simulink model "ValidateROM_PMSM"  (R2026a)
settings: Solver=FixedStepAuto  StartTime=0  StopTime=5000  FixedStep=0.5
PreLoadFcn:
  | % Load the Test data set for verification
  | load Data/pmsm_temperature_data_large.mat;
  | 
  | % Picking up a test profile for verification
  | TestSet = timetables{57};
  | 
  | % Seperate the predictors and the response
  | TestSet_Predict = TestSet(:,1:7);
  | TestSet_Response = TestSet(:,8:11);
  | 
  | % Clear the original data to avoid duplication
  | clear TestSet;
  | clear timetables;
  | 
  | % Load the trained LSTM and NSS Model
  | load Models/LSTMTrainingOutput.mat
  | load Models/NSSTrainingOutput.mat
  | 
  | % Extract the corresponding input normalizations
  | meanX_lstm = LSTMtrainingOutput.Normalization.Mu{1,1:7};
  | stdX_lstm = LSTMtrainingOutput.Normalization.Sigma{1,1:7};
  | 
  | meanX_nss = NSStrainingOutput.Normalization.Mu{1,1:7};
  | stdX_nss = NSStrainingOutput.Normalization.Sigma{1,1:7};
  | 
  | 
  | % Extract output normalization
  | meanY_lstm = LSTMtrainingOutput.Normalization.Mu{1,8:11};
  | stdY_lstm = LSTMtrainingOutput.Normalization.Sigma{1,8:11};
  | 
  | meanY_nss = NSStrainingOutput.Normalization.Mu{1,[8:11]};
  | stdY_nss = NSStrainingOutput.Normalization.Sigma{1,[8:11]};
  | 
  | %meanY_nss = NSStrainingOutput.Normalization.Mu{1,[8 11 14 17]};
  | %stdY_nss = NSStrainingOutput.Normalization.Sigma{1,[8 11 14 17]};
  | 
  | % [-1.4912 0 0 -1.0704 0 0 -1.2954 0 0 -1.3511 0 0]
model workspace (MAT data in the model file):
  time = -1
values from neighbouring files (symbols this model uses):
  NSStrainingOutput =     [NSSTrainingOutput.mat]
libraries: deeplib x1, slident x1
settings Model: Creator=skeshavm  LastModifiedBy=msatra
settings DataIOCC: SaveFormat=StructureWithTime
settings OptimizationCC: UseDivisionForNetSlopeComputation=on  GainParamInheritBuiltInType=on  UseFloatMulNetSlope=on  InlineInvariantSignals=on  StrengthReduction=on  PassReuseOutputArgsThreshold=0.0  InitFltsAndDblsToZero=on  EfficientFloat2IntCast=on  OptimizationPriority=Speed  MultiThreadedLoops=on  AutoScheduleForLoops=on  UseRestrictQualifier=on  DenormalBehavior=FlushToZero
settings DebuggingCC: InheritedTsInSrcMsg=none  MultiTaskCondExecSysMsg=none  MultiTaskRateTransMsg=warning
settings HardwareCC: TargetLongLongMode=on
settings SFSimCC: SimTargetLang=C++
settings RTWCC: Toolchain=Microsoft Visual C++ 2019 v16.0 | nmake (64-bit Windows)  BuildConfiguration=Faster Runs  TargetLang=C++  CheckMdlBeforeBuild=Warning  GPUErrorChecks=on  GPUComputeCapability=7.5
settings GRTTargetCC: TargetLangStandard=C++11 (ISO)  CodeInterfacePackaging=C++ class

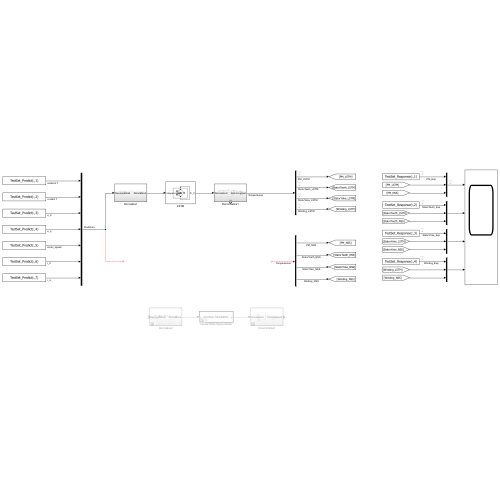
[thumbnail: Simulink's stored preview of the top-level diagram]
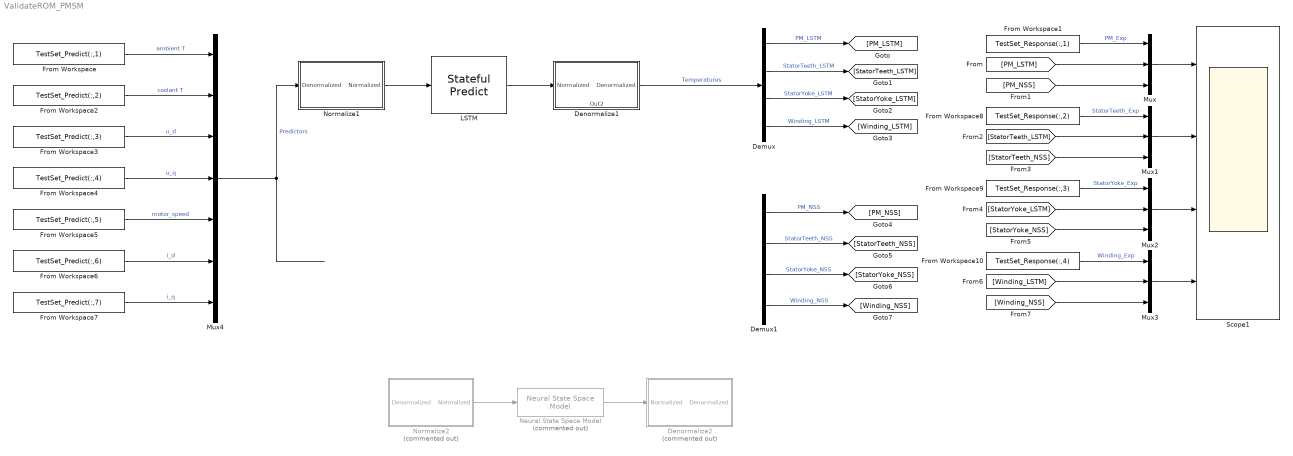
== system ValidateROM_PMSM ==
  Demux : Demux
  Demux1 : Demux
  Denormalize1 : Subsystem
      settings: PortSchema="{\"entries\":[{\"content\":{\"sides\":[{\"content\":{\"connectorIds\":[\"In1\"]},\"type\":\"ConnectorPlacement.EquallySpacedRectSide\",\"uuid\":\"378bcf4c-6683-4062-ab7f-3d581c01bba9\"},{\"content\":{\"connectorIds\":[\"Out1\"],\"side\":\"RIGHT\"},\"type\":\"ConnectorPlacement.EquallySpacedRectSide\",\"uuid\":\"d50369fd-00a0-4fa4-8ce4-c1bc44e9feeb\"},{\"content\":{\"side\":\"TOP\"},\"type\":\"ConnectorPlacement.EquallySpacedRectSide\",\"uuid\":\"bbe2daf0-7cf2-4950-af80-cb885b06a7dc\"},{\"content\":{\"connectorIds\":[\"Out2\"],\"side\":\"BOTTOM\"},\"type\":\"ConnectorPlacement.EquallySpacedRectSide\",\"uuid\":\"6647e6bb-1933-4f5d-ba46-5deef3c85e19\"}]},\"type\":\"ConnectorPlacement.EquallySpacedConnector\",\"uuid\":\"4ece9d1b-3b81-464e-b5f8-e83b248e3e90\"}],\"packageUris\":[\"http://schema.mathworks.com/mf0/Connector/R2020b\"],\"version\":\"1.0\"}"
  Denormalize2 : Subsystem  Commented=on
  From Workspace : FromWorkspace  VariableName=TestSet_Predict(:,1)
  From Workspace1 : FromWorkspace  VariableName=TestSet_Response(:,1)  SampleTime=5
  From Workspace10 : FromWorkspace  VariableName=TestSet_Response(:,4)  SampleTime=5
  From Workspace2 : FromWorkspace  VariableName=TestSet_Predict(:,2)
  From Workspace3 : FromWorkspace  VariableName=TestSet_Predict(:,3)
  From Workspace4 : FromWorkspace  VariableName=TestSet_Predict(:,4)
  From Workspace5 : FromWorkspace  VariableName=TestSet_Predict(:,5)
  From Workspace6 : FromWorkspace  VariableName=TestSet_Predict(:,6)
  From Workspace7 : FromWorkspace  VariableName=TestSet_Predict(:,7)
  From Workspace8 : FromWorkspace  VariableName=TestSet_Response(:,2)  SampleTime=5
  From Workspace9 : FromWorkspace  VariableName=TestSet_Response(:,3)  SampleTime=5
  LSTM : deeplib/Stateful Predict  Network=Network from MAT-file  NetworkFunction=untitled  NetworkFilePath=Models\LSTMTrainingNetwork.mat  SimulateUsing=Auto mode  InputDataFormats={ 'sequenceinput', 'CBT' }  SampleTime=0.5  ForceInterpretedSim=off  EnableDLNetwork=on  LastKnownNetworkFilePath=''  LastKnownNetworkTimeStamp=''
  Mux{,1..3} (4 alike) : Mux  Inputs=3
  Mux4 : Mux  Inputs=7
  Neural State Space Model : slident/Models/Neural State Space Model  Commented=on  sys=NSStrainingOutput.NSSModel  x0type=internal  ic=[-1.4912 -1.0704 -1.2954 -1.3511]  returnx=off  returndx=off
  Normalize1 : Subsystem
  Normalize2 : Subsystem  Commented=on
  Scope1 : Scope  NumInputPorts=4
      settings: ActiveDisplayYMinimum=21.188522711990892  ActiveDisplayYMaximum=80.175708667038492
  wires:
  Demux/2 -> [StatorTeeth_LSTM]  "StatorTeeth_LSTM"
  Demux/3 -> [StatorYoke_LSTM]  "StatorYoke_LSTM"
  Mux4/1 -> Normalize1/1(Denormalized)  "Predictors"
  Demux/4 -> [Winding_LSTM]  "Winding_LSTM"
  Demux/1 -> [PM_LSTM]  "PM_LSTM"
  Normalize1/1(Normalized) -> LSTM/1
  Denormalize1/1(Denormalized) -> Demux/1  "Temperatures"
  Mux1/1 -> Scope1/2
  Mux2/1 -> Scope1/3
  Mux3/1 -> Scope1/4
  From Workspace1/1 -> Mux/1  "PM_Exp"
  From Workspace8/1 -> Mux1/1  "StatorTeeth_Exp"
  From Workspace9/1 -> Mux2/1  "StatorYoke_Exp"
  From Workspace10/1 -> Mux3/1  "Winding_Exp"
  From Workspace/1 -> Mux4/1  "ambient T"
  From Workspace2/1 -> Mux4/2  "coolant T"
  From Workspace3/1 -> Mux4/3  "u_d"
  From Workspace4/1 -> Mux4/4  "u_q"
  From Workspace5/1 -> Mux4/5  "motor_speed"
  From Workspace6/1 -> Mux4/6  "i_d"
  From Workspace7/1 -> Mux4/7  "i_q"
  Mux/1 -> Scope1/1
  LSTM/1 -> Denormalize1/1(Normalized)
  Neural State Space Model/1 -> Denormalize2/1(Normalized)
  Normalize2/1(Normalized) -> Neural State Space Model/1
  Demux1/1 -> [PM_NSS]  "PM_NSS"
  Demux1/2 -> [StatorTeeth_NSS]  "StatorTeeth_NSS"
  Demux1/3 -> [StatorYoke_NSS]  "StatorYoke_NSS"
  Demux1/4 -> [Winding_NSS]  "Winding_NSS"
  [PM_LSTM] -> Mux/2
  [PM_NSS] -> Mux/3
  [StatorTeeth_LSTM] -> Mux1/2
  [StatorTeeth_NSS] -> Mux1/3
  [StatorYoke_LSTM] -> Mux2/2
  [StatorYoke_NSS] -> Mux2/3
  [Winding_LSTM] -> Mux3/2
  [Winding_NSS] -> Mux3/3
  ? -> Demux1/1  "Temperatures"

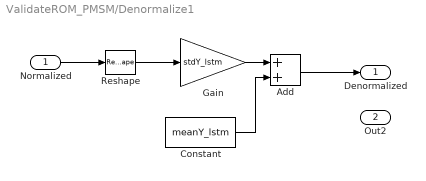
== system ValidateROM_PMSM/Denormalize1 ==
  Normalized : Inport
  Add : Sum
  Constant : Constant  Value=meanY_lstm
  Gain : Gain  Gain=stdY_lstm  OutDataTypeStr=single
  Reshape : Reshape
  Denormalized : Outport
  Out2 : Outport  Port=2
  wires:
  Normalized/1 -> Reshape/1
  Add/1 -> Denormalized/1
  Gain/1 -> Add/1
  Constant/1 -> Add/2
  Reshape/1 -> Gain/1

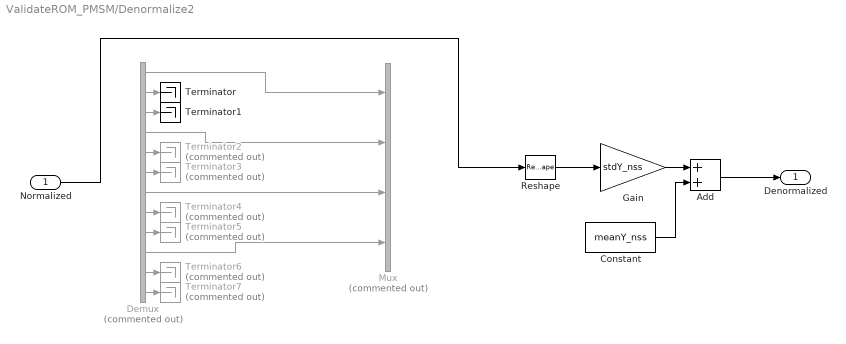
== system ValidateROM_PMSM/Denormalize2 ==
  Normalized : Inport
  Add : Sum
  Constant : Constant  Value=meanY_nss
  Demux : Demux  Commented=on  Outputs=12
  Gain : Gain  Gain=stdY_nss  OutDataTypeStr=single
  Mux : Mux  Commented=on
  Reshape : Reshape
  Terminator : Terminator
  Terminator1 : Terminator
  Terminator{2..7} (6 alike) : Terminator  Commented=on
  Denormalized : Outport
  wires:
  Reshape/1 -> Gain/1
  Constant/1 -> Add/2
  Gain/1 -> Add/1
  Add/1 -> Denormalized/1
  Normalized/1 -> Reshape/1
  Demux/1 -> Mux/1
  Demux/4 -> Mux/2
  Demux/7 -> Mux/3
  Demux/10 -> Mux/4
  Demux/2 -> Terminator/1
  Demux/3 -> Terminator1/1
  Demux/5 -> Terminator2/1
  Demux/6 -> Terminator3/1
  Demux/8 -> Terminator4/1
  Demux/9 -> Terminator5/1
  Demux/11 -> Terminator6/1
  Demux/12 -> Terminator7/1

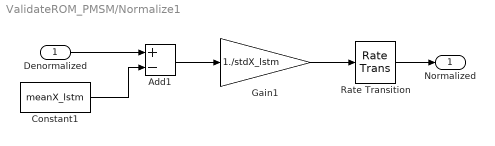
== system ValidateROM_PMSM/Normalize1 ==
  Denormalized : Inport
  Add1 : Sum  Inputs=+-
  Constant1 : Constant  Value=meanX_lstm
  Gain1 : Gain  Gain=1./stdX_lstm
  Rate Transition : RateTransition
  Normalized : Outport
  wires:
  Denormalized/1 -> Add1/1
  Constant1/1 -> Add1/2
  Add1/1 -> Gain1/1
  Gain1/1 -> Rate Transition/1
  Rate Transition/1 -> Normalized/1

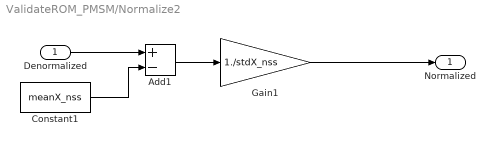
== system ValidateROM_PMSM/Normalize2 ==
  Denormalized : Inport
  Add1 : Sum  Inputs=+-
  Constant1 : Constant  Value=meanX_nss
  Gain1 : Gain  Gain=1./stdX_nss
  Normalized : Outport
  wires:
  Gain1/1 -> Normalized/1
  Add1/1 -> Gain1/1
  Constant1/1 -> Add1/2
  Denormalized/1 -> Add1/1
